simulink library "DHW_Energy_Tapping"  (Simulink 7.6)
settings: Solver=ode45  StartTime=0.0  StopTime=10.0  RelTol=1e-3
settings Model: Creator=lena.frank  LastModifiedBy=drhf

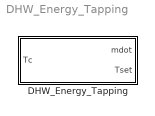
== system DHW_Energy_Tapping ==
  DHW_Energy_Tapping : Subsystem  mask{mdot_nom=1/60, times=[7     7.1 7.5   8.083 8.25  8.5   8.75  9     9.5   10.5  11.5  11.75 12.75 14.5  15.5  16.5  18    18.25 18.5  19    20.5  21.25 21.5]*3600, energies=[0.105 1.4 0.105 0.105 0.105 0.105 0.105 0.105 0.105 0.105 0.105 0.105 0.315 0.105 0.105 0.105 0.105 0.105 0.105 0.105 0.735 0.105 1.4 ]*36e5, dT_set=[30    30  30    30    30    30    30    30    30    30    30    30    45    30    30    30    30    30    30    30    45    30    30  ], coeffs=[3     6   3     3     3     3     3     3     3     3     3     3     4     3     3     3     3     3     3     3     4     3     6   ]}
      mask prompts: mdot_nom "nominal massflow [kg/s]"; times "vector of start times of taps [s]"; energies "vector of energies of taps [J]"; dT_set "vector of delta set temperatures of taps [K]"; coeffs "vector of coefficients of nominal massflow of taps [-]"
      mask Display: disp('dhw_EN13203')

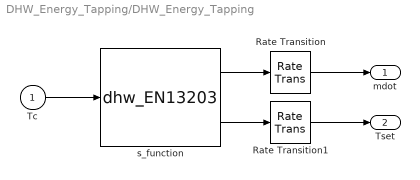
== system DHW_Energy_Tapping/DHW_Energy_Tapping ==
  Tc : Inport
  Rate Transition : RateTransition
  Rate Transition1 : RateTransition
  s_function : S-Function  FunctionName=dhw_EN13203  Parameters=times,energies,coeffs,dT_set,mdot_nom  EnableBusSupport=off
  mdot : Outport
  Tset : Outport  Port=2
  wires:
  s_function/2 -> Rate Transition1/1
  s_function/1 -> Rate Transition/1
  Tc/1 -> s_function/1
  Rate Transition/1 -> mdot/1
  Rate Transition1/1 -> Tset/1
